simulink model "x4DOF_Model"  (R2023a)
settings: Solver=VariableStepAuto  StartTime=0.0  StopTime=15  RelTol=1e-3
InitFcn:
  | data = readtable("car_rig_data.xlsx");
undefined symbols (not defined in the file): C_matrix_subbed, Init_param, Init_param_dot, K_matrix_subbed, M_matrix_subbed
settings Model: Creator=Sebastian  LastModifiedBy=Sebastian
settings DataIOCC: ExternalInput=m_mat,k_mat,c_mat

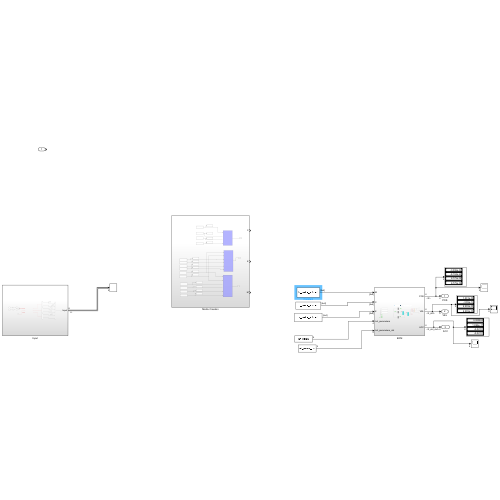
[thumbnail: Simulink's stored preview of the top-level diagram]
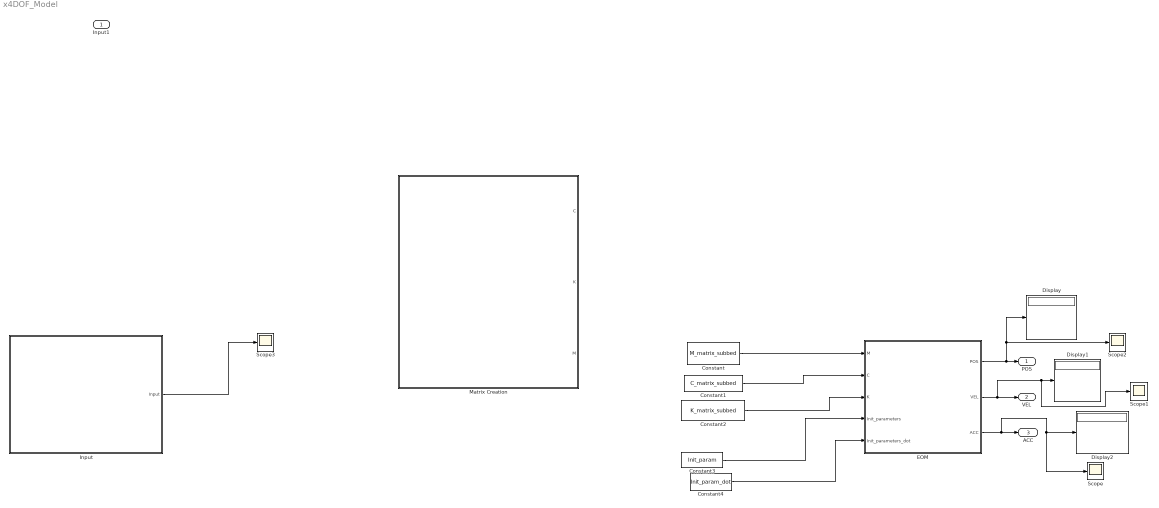
== system x4DOF_Model ==
  Input1 : Inport
  Constant : Constant  Value=M_matrix_subbed
  Constant1 : Constant  Value=C_matrix_subbed
  Constant2 : Constant  Value=K_matrix_subbed
  Constant3 : Constant  Value=Init_param
  Constant4 : Constant  Value=Init_param_dot
  Display : Display
  Display1 : Display
  Display2 : Display
  EOM : Subsystem
  Input : Subsystem
  Matrix Creation : Subsystem
  Scope{,1..3} (4 alike) : Scope
  POS : Outport
  VEL : Outport  Port=2
  ACC : Outport  Port=3
  wires:
  EOM/1(POS) -> Scope2/1, Display/1, POS/1
  EOM/2(VEL) -> Scope1/1, Display1/1, VEL/1
  EOM/3(ACC) -> Scope/1, Display2/1, ACC/1
  Input/1(Input) -> Scope3/1
  Constant/1 -> EOM/1(M)
  Constant1/1 -> EOM/2(C)
  Constant2/1 -> EOM/3(K)
  Constant3/1 -> EOM/4(Init_parameters)
  Constant4/1 -> EOM/5(Init_parameters_dot)

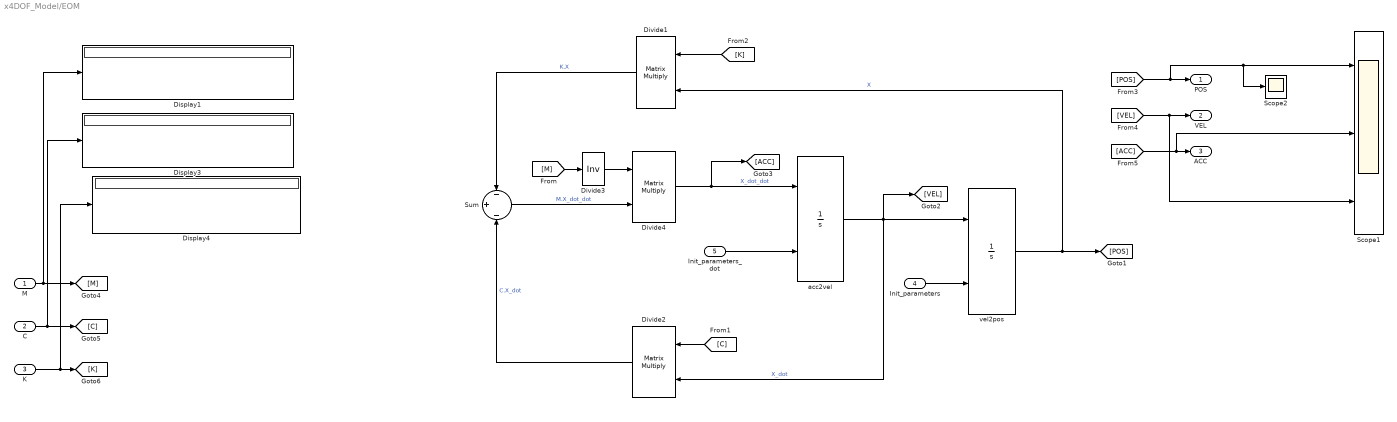
== system x4DOF_Model/EOM ==
  M : Inport
  C : Inport  Port=2
  K : Inport  Port=3
  Init_parameters : Inport  Port=4
  Init_parameters_dot : Inport  Port=5
  Display1 : Display
  Display3 : Display
  Display4 : Display
  Divide1 : Product  Multiplication=Matrix(*)
  Divide2 : Product  Multiplication=Matrix(*)
  Divide3 : Product  Inputs=/  Multiplication=Matrix(*)
  Divide4 : Product  Multiplication=Matrix(*)
  Scope1 : Scope  NumInputPorts=3
  Scope2 : Scope
  Sum : Sum  Inputs=-|+|-
  acc2vel : Integrator  InitialConditionSource=external
  vel2pos : Integrator  InitialConditionSource=external
  POS : Outport
  VEL : Outport  Port=2
  ACC : Outport  Port=3
  wires:
  Divide4/1 -> [ACC], acc2vel/1  "X_dot_dot"
  [C] -> Divide2/1
  vel2pos/1 -> [POS], Divide1/2  "X"
  Divide1/1 -> Sum/1  "K.X"
  acc2vel/1 -> vel2pos/1, [VEL], Divide2/2  "X_dot"
  [K] -> Divide1/1
  C/1 -> Display3/1, [C]
  [ACC] -> Scope1/2, ACC/1
  [M] -> Divide3/1
  [VEL] -> Scope1/3, VEL/1
  Sum/1 -> Divide4/2  "M.X_dot_dot"
  Divide2/1 -> Sum/3  "C.X_dot"
  Divide3/1 -> Divide4/1
  [POS] -> Scope2/1, Scope1/1, POS/1
  M/1 -> Display1/1, [M]
  K/1 -> Display4/1, [K]
  Init_parameters_dot/1 -> acc2vel/2
  Init_parameters/1 -> vel2pos/2

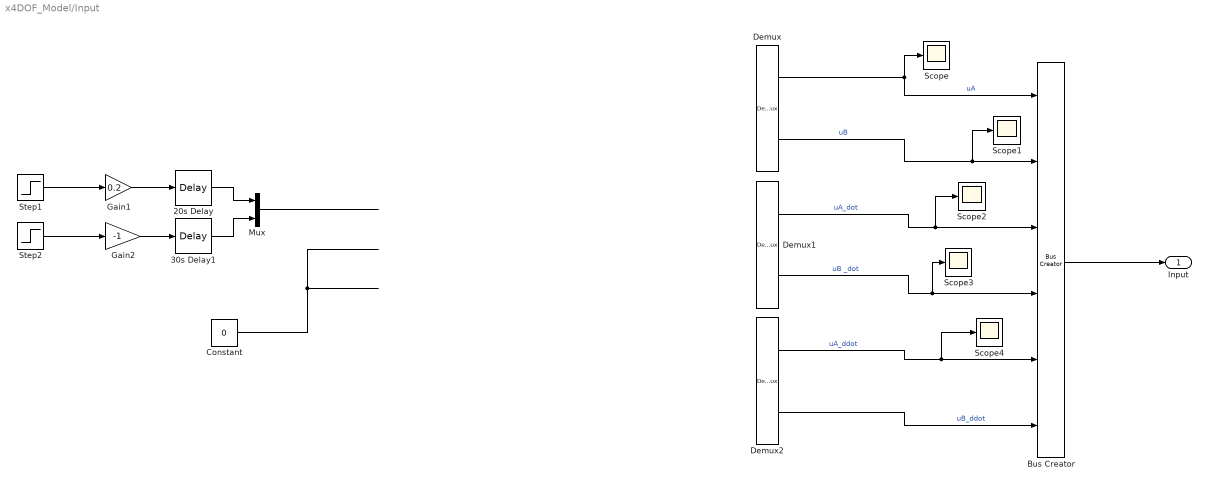
== system x4DOF_Model/Input ==
  20s Delay : TransportDelay  DelayTime=20
  30s Delay1 : TransportDelay  DelayTime=30
  Bus Creator : BusCreator  Inputs=6
  Constant : Constant  Value=0
  Demux : Demux  Outputs=2
  Demux1 : Demux  Outputs=2
  Demux2 : Demux  Outputs=2
  Gain1 : Gain  Gain=0.2
  Gain2 : Gain  Gain=-1
  Mux : Mux  Inputs=2
  Scope{,1..4} (5 alike) : Scope
  Step1 : Step  SampleTime=0
  Step2 : Step  SampleTime=0
  Input : Outport
  wires:
  Mux/1 -> ?
  Constant/1 -> ?
  ? -> Demux/1  "U_filt"
  ? -> Demux1/1  "U_dot_filt"
  ? -> Demux2/1
  Step2/1 -> Gain2/1
  Step1/1 -> Gain1/1
  Gain1/1 -> 20s Delay/1
  Gain2/1 -> 30s Delay1/1
  20s Delay/1 -> Mux/1
  30s Delay1/1 -> Mux/2
  Demux/1 -> Scope/1, Bus Creator/1  "uA"
  Demux/2 -> Bus Creator/2, Scope1/1  "uB"
  Demux1/1 -> Scope2/1, Bus Creator/3  "uA_dot"
  Demux1/2 -> Scope3/1, Bus Creator/4  "uB _dot"
  Demux2/1 -> Scope4/1, Bus Creator/5  "uA_ddot"
  Demux2/2 -> Bus Creator/6  "uB_ddot"
  Bus Creator/1 -> Input/1

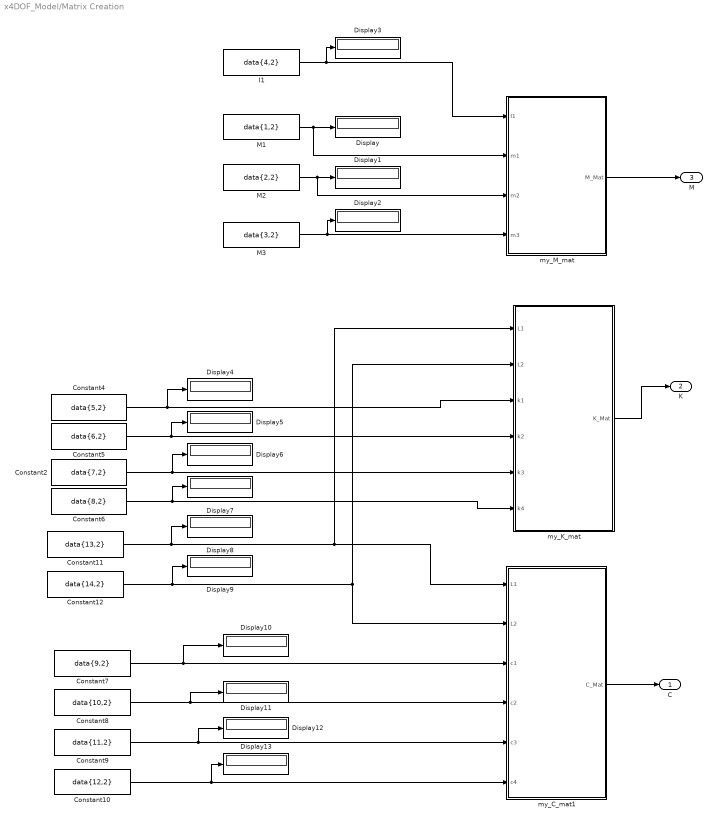
== system x4DOF_Model/Matrix Creation ==
  Constant10 : Constant  Value=data{12,2}
  Constant11 : Constant  Value=data{13,2}
  Constant12 : Constant  Value=data{14,2}
  Constant2 : Constant  Value=data{7,2}
  Constant4 : Constant  Value=data{5,2}
  Constant5 : Constant  Value=data{6,2}
  Constant6 : Constant  Value=data{8,2}
  Constant7 : Constant  Value=data{9,2}
  Constant8 : Constant  Value=data{10,2}
  Constant9 : Constant  Value=data{11,2}
  Display{,1..13} (14 alike) : Display
  I1 : Constant  Value=data{4,2}
  M1 : Constant  Value=data{1,2}
  M2 : Constant  Value=data{2,2}
  M3 : Constant  Value=data{3,2}
  my_C_mat1 : MATLAB Function  TreatAsAtomicUnit=on
  my_K_mat : MATLAB Function  TreatAsAtomicUnit=on
  my_M_mat : MATLAB Function  TreatAsAtomicUnit=on
  C : Outport
  K : Outport  Port=2
  M : Outport  Port=3
  wires:
  my_C_mat1/1(C_Mat) -> C/1
  my_K_mat/1(K_Mat) -> K/1
  my_M_mat/1(M_Mat) -> M/1
  M1/1 -> my_M_mat/2(m1), Display/1
  M2/1 -> my_M_mat/3(m2), Display1/1
  I1/1 -> Display3/1, my_M_mat/1(I1)
  M3/1 -> Display2/1, my_M_mat/4(m3)
  Constant5/1 -> Display5/1, my_K_mat/4(k2)
  Constant2/1 -> Display6/1, my_K_mat/5(k3)
  Constant6/1 -> Display7/1, my_K_mat/6(k4)
  Constant10/1 -> Display13/1, my_C_mat1/6(c4)
  Constant8/1 -> Display11/1, my_C_mat1/4(c2)
  Constant7/1 -> Display10/1, my_C_mat1/3(c1)
  Constant11/1 -> Display8/1, my_K_mat/1(L1), my_C_mat1/1(L1)
  Constant12/1 -> Display9/1, my_K_mat/2(L2), my_C_mat1/2(L2)
  Constant4/1 -> Display4/1, my_K_mat/3(k1)
  Constant9/1 -> Display12/1, my_C_mat1/5(c3)

== matlab function x4DOF_Model/Matrix Creation/my_K_mat ==
  data: L1 input; K_Mat output; L2 input; k1 input; k2 input; k3 input; k4 input
function K_Mat = my_K_mat(L1,L2,k1,k2,k3,k4)
%#codegen

%    This function was generated by the Symbolic Math Toolbox version 9.3.
%    06-Jun-2023 14:11:42

% L1 = complex(L1);  % if required to enforce complex operations
% L2 = complex(L2);  % if required to enforce complex operations
% k1 = complex(k1);  % if required to enforce complex operations
% k2 = complex(k2);  % if required to enforce complex operations
% k3 = complex(k3);  % if required to enforce complex operations
% k4 = complex(k4);  % if required to enforce complex operations
t2 = L1.*k1;
t3 = L2.*k2;
t4 = -k1;
t5 = -k2;
t6 = -t2;
t7 = -t3;
t8 = t3+t6;
K_Mat = reshape([k1+k2,t8,t4,t5,t8,L1.*t2+L2.*t3,t2,t7,t4,t2,k1+k3,0.0,t5,t7,0.0,k2+k4],[4,4]);
end

== matlab function x4DOF_Model/Matrix Creation/my_M_mat ==
  data: I1 input; M_Mat output; m1 input; m2 input; m3 input
function M_Mat = my_M_mat(I1,m1,m2,m3)
%#codegen

%    This function was generated by the Symbolic Math Toolbox version 9.3.
%    06-Jun-2023 14:11:41

% I1 = complex(I1);  % if required to enforce complex operations
% m1 = complex(m1);  % if required to enforce complex operations
% m2 = complex(m2);  % if required to enforce complex operations
% m3 = complex(m3);  % if required to enforce complex operations
M_Mat = reshape([m1,0.0,0.0,0.0,0.0,I1,0.0,0.0,0.0,0.0,m2,0.0,0.0,0.0,0.0,m3],[4,4]);
end

== matlab function x4DOF_Model/Matrix Creation/my_C_mat1 ==
  data: L1 input; C_Mat output; L2 input; c1 input; c2 input; c3 input; c4 input
function C_Mat = my_C_mat(L1,L2,c1,c2,c3,c4)
%#codegen

%    This function was generated by the Symbolic Math Toolbox version 9.3.
%    06-Jun-2023 14:11:42

% L1 = complex(L1);  % if required to enforce complex operations
% L2 = complex(L2);  % if required to enforce complex operations
% c1 = complex(c1);  % if required to enforce complex operations
% c2 = complex(c2);  % if required to enforce complex operations
% c3 = complex(c3);  % if required to enforce complex operations
% c4 = complex(c4);  % if required to enforce complex operations
t2 = L1.*c1;
t3 = L2.*c2;
t4 = -c1;
t5 = -c2;
t6 = -t2;
t7 = -t3;
t8 = t3+t6;
C_Mat = reshape([c1+c2,t8,t4,t5,t8,L1.*t2+L2.*t3,t2,t7,t4,t2,c1+c3,0.0,t5,t7,0.0,c2+c4],[4,4]);
end
